simulink model "test_no_ctrl"  (R2021b)
settings: Solver=VariableStepAuto  StartTime=0.0  StopTime=600  RelTol=1e-3
values from neighbouring files (symbols this model uses):
  floor_height = 3    [load_data.m]
  gearbox = 1    [load_data.m]
  Rp = 0.5    [load_data.m]
  Ts = 1e-3    (= 0.001)    [load_data.m]
libraries: LiftMotionControlLibrary x5
settings Model: Creator=manue  LastModifiedBy=manue
settings ConfigComp: PLC_TargetIDE=generic  PLC_MultiTBSigbuilderTimeRange=off  PLC_InlineEnumCastFunction=off

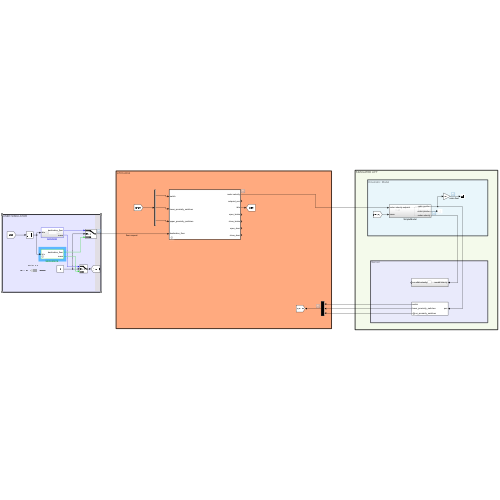
[thumbnail: Simulink's stored preview of the top-level diagram]
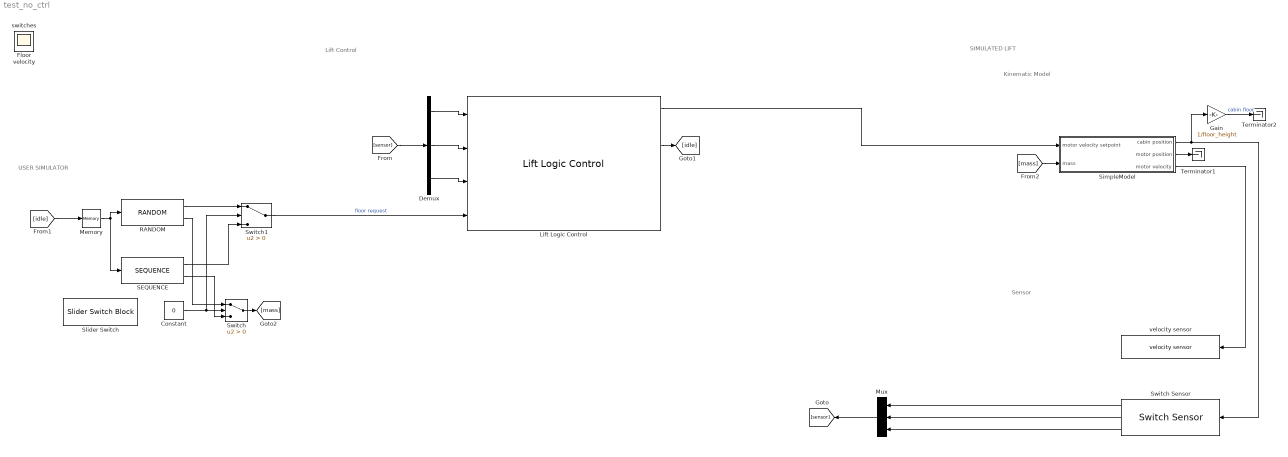
== system test_no_ctrl ==
  note: SIMULATED LIFT
  note: USER SIMULATOR
  note: Sensor
  note: Kinematic Model
  note: Lift Control
  Constant : Constant  Value=0
  Demux : Demux  Outputs=3
  Gain : Gain  Gain=1/floor_height
  Lift Logic Control : LiftMotionControlLibrary/Lift Logic Control  floor_height=floor_height  num_floors=num_floors  cabin_height=cabin_height  proximity_distance=proximity_distance  MinVel=MinVel  MaxVel=MaxVel  Ts=Ts  MaxAcc=MaxAcc  MaxJerk=MaxJerk  gearbox=gearbox  cabin_offset=cabin_offset  Rp=Rp  motion_profile=Profile 1: single speed  waiting_time_open_door=waiting_time_open_door  waiting_time_close_door=waiting_time_close_door  waiting_time_open_brake=waiting_time_open_brake  waiting_time_close_brake_copy=waiting_time_close_brake  waiting_time_steady_state=waiting_time_steady_state
  Memory : Memory
  Mux : Mux  Inputs=3
  "RANDOM " : LiftMotionControlLibrary/RANDOM  SystemSampleTime=-1  VariantActivationTime=update diagram  Latency=0  AutoFrameSizeCalculation=off
  "SEQUENCE " : LiftMotionControlLibrary/SEQUENCE  sequence=[10 5 10 15]
  SimpleModel : Subsystem
  Slider Switch : SliderSwitchBlock
      settings: Values={{'SEQUENCE', 'RANDOM'}, [0 1]}
  Switch : Switch  Criteria=u2 > Threshold
  Switch Sensor : LiftMotionControlLibrary/Switch Sensor  floor_height=floor_height  num_floors=num_floors  proximity_distance=proximity_distance  cabin_height=cabin_height
  Switch1 : Switch  Criteria=u2 > Threshold
  Terminator1 : Terminator
  Terminator2 : Terminator
  velocity sensor : LiftMotionControlLibrary/velocity sensor  SystemSampleTime=-1  VariantActivationTime=update diagram  Latency=0  AutoFrameSizeCalculation=off
  Floor : Scope
  switches : Scope
  velocity : Scope
  wires:
  Switch1/1 -> Lift Logic Control/4  "floor request"
  SimpleModel/1(cabin position) -> Gain/1, Switch Sensor/1
  Switch Sensor/1 -> Mux/1
  Switch Sensor/2 -> Mux/2
  Switch Sensor/3 -> Mux/3
  Demux/3 -> Lift Logic Control/3
  Demux/2 -> Lift Logic Control/2
  Demux/1 -> Lift Logic Control/1
  Mux/1 -> [sensor]
  [sensor] -> Demux/1
  SimpleModel/2(motor position) -> Terminator1/1
  Lift Logic Control/1 -> SimpleModel/1(motor velocity setpoint)
  Lift Logic Control/3 -> [idle]
  "RANDOM "/2 -> Switch/1
  [mass] -> SimpleModel/2(mass)
  [idle] -> Memory/1
  Memory/1 -> "SEQUENCE "/1, "RANDOM "/1
  SimpleModel/3(motor velocity) -> velocity sensor/1
  Gain/1 -> Terminator2/1  "cabin floor"
  "SEQUENCE "/2 -> Switch/3
  Switch/1 -> [mass]
  "RANDOM "/1 -> Switch1/1
  "SEQUENCE "/1 -> Switch1/3
  Constant/1 -> Switch1/2, Switch/2

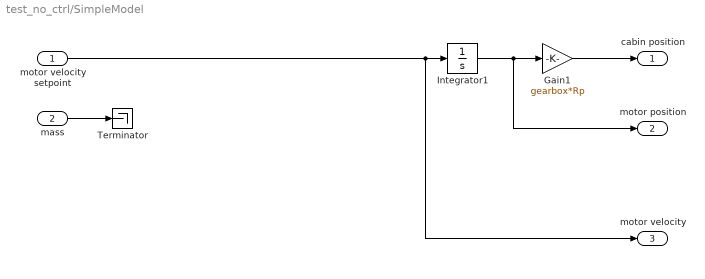
== system test_no_ctrl/SimpleModel ==
  motor velocity setpoint : Inport
  mass : Inport  Port=2
  Gain1 : Gain  Gain=gearbox*Rp
  Integrator1 : Integrator
  Terminator : Terminator
  cabin position : Outport
  motor position : Outport  Port=2
  motor velocity : Outport  Port=3
  wires:
  motor velocity setpoint/1 -> motor velocity/1, Integrator1/1
  Integrator1/1 -> motor position/1, Gain1/1
  Gain1/1 -> cabin position/1
  mass/1 -> Terminator/1
